simulink model "Comparatie_estimator_cu_simplu"  (R2023b)
settings: Solver=VariableStepAuto  StartTime=0.0  StopTime=100  RelTol=1e-3
values from neighbouring files (symbols this model uses):
  A = [0 lambda 0 0 ... (first row only)    [rotary_inverted_pendulum.m]    (also in sis_liniar.m)
  B = [0; B21; 0; B41]./lambda    [rotary_inverted_pendulum.m]    (also in sis_liniar.m)
  C = [0 0 1 0]    [rotary_inverted_pendulum.m]
  K = lqr(A,B,Q,R)    [rotary_inverted_pendulum.m]
  N = -inv(C*inv(A-B*K)*B)    [rotary_inverted_pendulum.m]
settings Model: Creator=ovidiuceoca  LastModifiedBy=ovidiuceoca

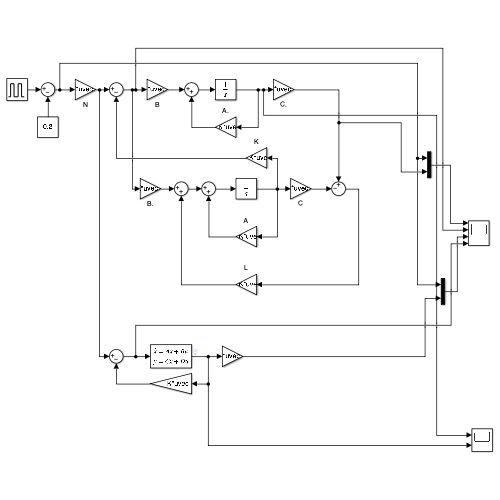
[thumbnail: Simulink's stored preview of the top-level diagram]
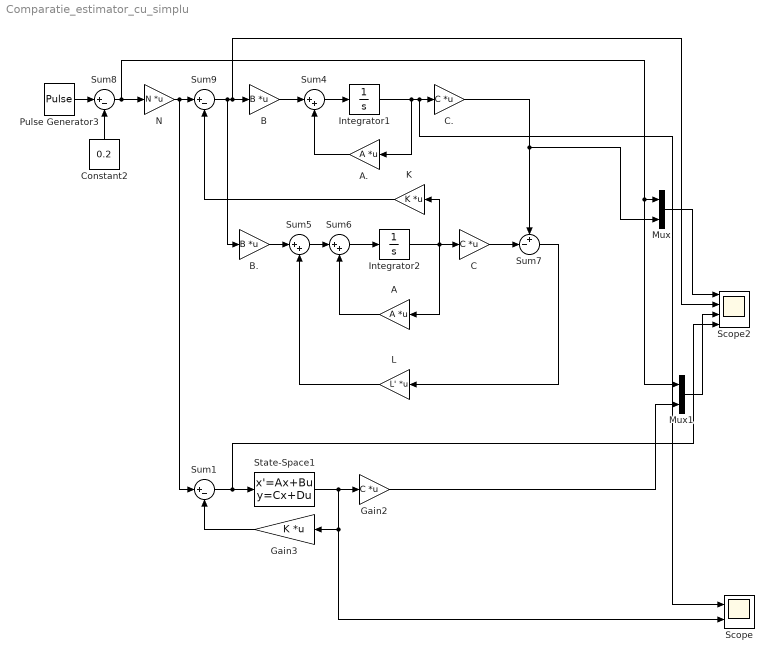
== system Comparatie_estimator_cu_simplu ==
  A : Gain  Gain=A  Multiplication=Matrix(K*u) (u vector)
  A. : Gain  Gain=A  Multiplication=Matrix(K*u) (u vector)
  B : Gain  Gain=B  Multiplication=Matrix(K*u) (u vector)
  B. : Gain  Gain=B  Multiplication=Matrix(K*u) (u vector)
  C : Gain  Gain=C  Multiplication=Matrix(K*u) (u vector)
  C. : Gain  Gain=C  Multiplication=Matrix(K*u) (u vector)
  Constant2 : Constant  Value=0.2
  Gain2 : Gain  Gain=C  Multiplication=Matrix(K*u) (u vector)
  Gain3 : Gain  Gain=K  Multiplication=Matrix(K*u) (u vector)
  Integrator1 : Integrator
  Integrator2 : Integrator  InitialCondition=[1,1,1,1]
  K : Gain  Gain=K  Multiplication=Matrix(K*u) (u vector)
  L : Gain  Gain=L'  Multiplication=Matrix(K*u) (u vector)
  Mux : Mux  Inputs=2
  Mux1 : Mux  Inputs=2
  N : Gain  Gain=N  Multiplication=Matrix(K*u) (u vector)
  Pulse Generator3 : DiscretePulseGenerator  PulseType=Time based  Amplitude=1.5  Period=30  PulseWidth=50  PhaseDelay=15
  Scope : Scope  NumInputPorts=2
  Scope2 : Scope  NumInputPorts=4
  State-Space1 : StateSpace  A=A  B=B  C=eye(4)  D=[0;0;0;0]  InitialCondition=[0;0;0;0]
  Sum1 : Sum  Inputs=|+-
  Sum4 : Sum  Inputs=|++
  Sum5 : Sum  Inputs=|++
  Sum6 : Sum  Inputs=|++
  Sum7 : Sum  Inputs=+-|
  Sum8 : Sum  Inputs=|+-
  Sum9 : Sum  Inputs=|+-
  wires:
  Gain2/1 -> Mux1/2
  Sum1/1 -> Scope2/4, State-Space1/1
  Gain3/1 -> Sum1/2
  Sum5/1 -> Sum6/1
  B/1 -> Sum4/1
  A./1 -> Sum4/2
  L/1 -> Sum5/2
  C./1 -> Mux/2, Sum7/1
  N/1 -> Sum1/1, Sum9/1
  B./1 -> Sum5/1
  K/1 -> Sum9/2
  Sum6/1 -> Integrator2/1
  Pulse Generator3/1 -> Sum8/1
  Constant2/1 -> Sum8/2
  Sum4/1 -> Integrator1/1
  Sum8/1 -> Mux1/1, Mux/1, N/1
  C/1 -> Sum7/2
  Sum9/1 -> B./1, Scope2/2, B/1
  Sum7/1 -> L/1
  Integrator2/1 -> K/1, C/1, A/1
  A/1 -> Sum6/2
  Mux/1 -> Scope2/1
  Mux1/1 -> Scope2/3
  State-Space1/1 -> Scope/2, Gain3/1, Gain2/1
  Integrator1/1 -> A./1, Scope/1, C./1
